simulink model "acausalFiltering_t6"  (R2012b)
settings: Solver=FixedStepDiscrete  StartTime=0.0  StopTime=10.0  FixedStep=0.001  RelTol=1e-3
undefined symbols (not defined in the file): dfilt
libraries: dspmlti4 x2, dsparch4 x2
settings Model: BufferReuse=off  Creator=gilja  LastModifiedBy=NPTL
settings SolverCC: EnableConcurrentExecution=on  ConcurrentTasks=on
settings DataIOCC: SaveOutput=off  SignalLogging=off  DSMLogging=off  SaveTime=off
settings OptimizationCC: InlineParams=on  InlineInvariantSignals=on  OptimizeBlockIOStorage=off  BufferReuse=off  ExpressionFolding=off  LocalBlockOutputs=off
settings HardwareCC: ProdIntDivRoundTo=Zero  ProdEndianess=LittleEndian  ProdHWDeviceType=Generic->32-bit x86 compatible
settings ModelReferenceCC: ModelReferenceMinAlgLoopOccurrences=on
settings RTWCC: SystemTargetFile=xpctarget.tlc  TemplateMakefile=xpc_default_tmf  Description=xPC Target  ProcessScript=xpctarget_make_rtw_hook  RTWCompilerOptimization=On
settings CodeAppCC: MaxIdLength=62
settings xpcTargetCC: TargetFcnLib=ansi_tfl_table_tmw.mat  CodeReplacementLibrary=XPC_BLAS  ParMdlRefBuildCompliant=on  ConcurrentExecutionCompliant=on  CombineSignalStateStructs=off  GRTInterface=on  xPCTaskExecutionProfile=on  xPCRL32EventNumber=5000  xPCisDownloadable=off  xPCLoadParamSetFile=off  xPCConcurrentTasks=off  xPCEnableSFAnimation=off

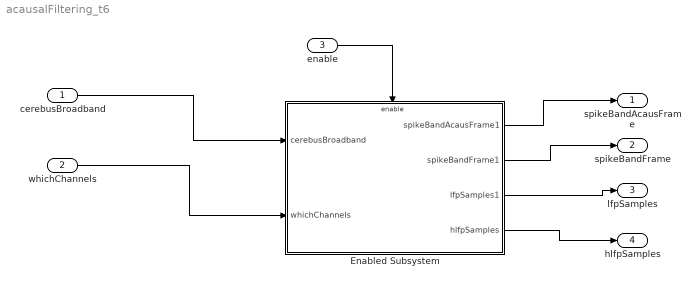
== system acausalFiltering_t6 ==
  cerebusBroadband : Inport  OutDataTypeStr=Bus: cerebusBroadband
  whichChannels : Inport  Port=2  PortDimensions=[1 32]
  enable : Inport  Port=3  OutDataTypeStr=uint8  PortDimensions=[1 1]
  Enabled Subsystem : Subsystem  TreatAsAtomicUnit=on
  spikeBandAcausFrame : Outport  BusOutputAsStruct=on
  spikeBandFrame : Outport  Port=2  BusOutputAsStruct=on
  lfpSamples : Outport  Port=3  BusOutputAsStruct=on
  hlfpSamples : Outport  Port=4  BusOutputAsStruct=on
  wires:
  cerebusBroadband/1 -> Enabled Subsystem/1(cerebusBroadband)
  whichChannels/1 -> Enabled Subsystem/2(whichChannels)
  enable/1 -> Enabled Subsystem/Enable
  Enabled Subsystem/1(spikeBandAcausFrame1) -> spikeBandAcausFrame/1
  Enabled Subsystem/2(spikeBandFrame1) -> spikeBandFrame/1
  Enabled Subsystem/3(lfpSamples1) -> lfpSamples/1
  Enabled Subsystem/4(hlfpSamples) -> hlfpSamples/1

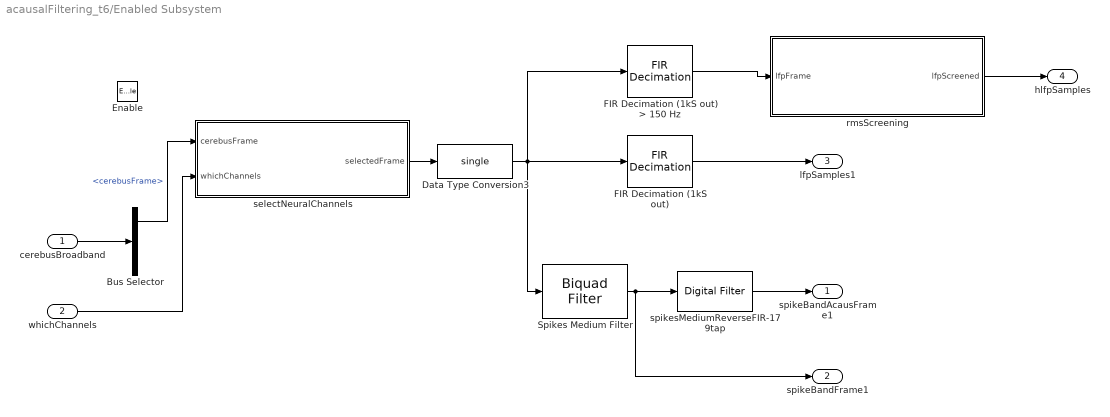
== system acausalFiltering_t6/Enabled Subsystem ==
  cerebusBroadband : Inport  OutDataTypeStr=Bus: cerebusBroadband
  whichChannels : Inport  Port=2  PortDimensions=[1 32]
  Enable : EnablePort
  Bus Selector : BusSelector  OutputSignals=cerebusFrame,outputValid,numDroppedUDPPackets
  Data Type Conversion3 : DataTypeConversion  OutDataTypeStr=single
  FIR Decimation (1kS out) : dspmlti4/FIR Decimation  h=fir1(360, 450/15000)  D=30  filtStruct=Direct form  framing=Enforce single-rate processing  inputOffset=0  outputBufInitCond=0  InputProcessing=Columns as channels (frame based)  firstCoeffDataTypeStr=Inherit: Same word length as input  firstCoeffLastDataTypeStr=Inherit: Same word length as input  firstCoeffMin=[]  firstCoeffMax=[]  outputDataTypeStr=Inherit: Same as accumulator  outputLastDataTypeStr=Inherit: Same as accumulator  outputMin=[]  outputMax=[]  roundingMode=Floor  overflowMode=off  FilterSource=Specify via dialog  FilterObject=Hm_firdecim
      settings: allowOverrides=off
  FIR Decimation (1kS out) > 150 Hz : dspmlti4/FIR Decimation  h=fir1(540, [150 450]/15000)  D=30  filtStruct=Direct form  framing=Enforce single-rate processing  inputOffset=0  outputBufInitCond=0  InputProcessing=Columns as channels (frame based)  firstCoeffDataTypeStr=Inherit: Same word length as input  firstCoeffLastDataTypeStr=Inherit: Same word length as input  firstCoeffMin=[]  firstCoeffMax=[]  outputDataTypeStr=Inherit: Same as accumulator  outputLastDataTypeStr=Inherit: Same as accumulator  outputMin=[]  outputMax=[]  roundingMode=Floor  overflowMode=off  FilterSource=Specify via dialog  FilterObject=Hm_firdecim
      settings: allowOverrides=off
  Spikes Medium Filter : dsparch4/Biquad Filter  IIRFiltStruct=Direct form II transposed  CoeffSource=Specify via dialog  BiQuadCoeffs="[0.95321773445431  -1.90644870937033 0.95323097500802 1 -1.90514144409761 0.90775595733389;  0.97970016700443  -1.95938672569874 0.97968655878878 1 -1.95804317832840 0.96073029104793]"  a0Flag=Warning  IC=0  ICnum=0  ICden=0  InputProcessing=Columns as channels (frame based)  denAccumFracLength=30  denProdOutputFracLength=30  secondMemoryFracLength=15  roundingMode=Floor  overflowMode=off  ScaleValues=1  optimizeScaleValues=on  ScaleValueMode=Specify via input port (g)  scaleValueFracLength=14  FilterSource=Specify via dialog  dfiltObjectName=dfilt.df2tsos([1 0.3 0.4],[1 0.1 0.2])
  rmsScreening : MATLAB Function  TreatAsAtomicUnit=on
  selectNeuralChannels : MATLAB Function  TreatAsAtomicUnit=on
  spikesMediumReverseFIR-179tap : dsparch4/Digital Filter  Tag=BlockMethodSubSystem  TypePopup=FIR (all zeros)  IIRFiltStruct=Direct form II transposed  AllPoleFiltStruct=Direct form  FIRFiltStruct=Direct form  CoeffSource=Specify via dialog  NumCoeffs=[0.00140028285573329 0.00145379314164095 0.00150549544372774 0.00155517517273179 0.00160261481898432 0.00164759444924944 0.00168989223087162 0.00172928498287283 0.00176554875356171 0.00179845942411888 0.00182779333752775 0.0018533279521235 0.00187484251893438 0.001892118781883 0.00190494169982069 0.00191310018925144 0.0019163878865113 0.00191460392804621 0.00190755374733714 0.00189504988690603 0.00187691282372934 0.0018529718062793 0.00182306570130567 0.00178704384836043 0.00174476691996755 0.00169610778522995 0.0016409523745676 0.00157920054317636 0.0015107669307024 0.00143558181452702 0.00135359195396933 0.00126476142262166 0.00116907242594854 0.00106652610119989 0.000957143296612834 0.000840965326803939 0.00071805470119018 0.000588495822216035 0.000452395650109955 0.000309884330846162 0.000161115783949557 6.26824674681641e-06 -0.000154455228359834 -0.000320826327031958 -0.000492591079996834 -0.000669469527359861 -0.000851155443662271 -0.00103731612710884 -0.00122759225635466 -0.0014215978181999 -0.00161892010950843 -0.00181911981658573 -0.00202173117519173 -0.0022262622142934 -0.00243219508655507 -0.00263898648845812 -0.00284606817285655 -0.00305284755660113 -0.00325870842577953 -0.00346301174092684 -0.00366509654442488 -0.0038642809721276 -0.00405986337106596 -0.00425112352489049 -0.00443732398850355 -0.0046177115331107 -0.00479151870268785 -0.00495796548265365 -0.00511626108120672 -0.00526560582364083 -0.00540519315955796 -0.00553421178272546 -0.00565184786295742 -0.00575728738913934 -0.00584971862221945 -0.00592833465663096 -0.00599233608834932 -0.00604093378741805 -0.00607335177246621 -0.00608883018440082 -0.00608662835612711 -0.00606602797479411 -0.00602633633273103 -0.00596688966289677 -0.00588705655431116 -0.00578624144260637 -0.00566388817048486 -0.00551948361255522 -0.00535256135864987 -0.00516270544943426 -0.00494955415778959 -0.00471280380912526 -0.00445221263349365 -0.00416760464208671 -0.00385887352039483 -0.00352598653007519 -0.00316898841130037 -0.00278800527713092 -0.00238324849124644 -0.00195501852016284 -0.00150370875087775 -0.00102980926475843 -0.000533910558313482 -1.6707201416282e-05 0.000520998576563121 0.00107829338229953 0.0016541492453484 0.00224742030589247 0.00285683961298849 0.0034810160428394 0.00411843134651596 0.00476743733644952 0.0054262532208052 0.00609296309471535 0.00676551359704508 0.00744171174116697 0.00811922292783734 0.0087955691479889 0.00946812738282926 0.010134128208247 0.0107906546100014 0.0114346410157853 0.0120628725495915 0.0126719845133399 0.0132584621000649 0.0138186403422851 0.0143487042986146 0.0148446894807868 0.015302482522666 0.0157178220919812 0.0160863000446657 0.0164033628209217 0.0166643130812326 0.0168643115796355 0.0169983792707087 0.0170613996457512 0.0170481212927745 0.0169531606738143 0.0167710051123323 0.0164960159823365 0.0161224320899623 0.0156443732373069 0.015055843957347 0.0143507374078498 0.0135228394112524 0.0125658326267011 0.0114733008394219 0.0102387333520141 0.00885552946126943 0.00731700300360289 0.0056163869514394 0.00374683804233694 0.00170144142218414 -0.000526784716648303 -0.00294488452160708 -0.00555995991030439 -0.00837916606463591 -0.0114097070082808 -0.0146588312871065 -0.0181338277715989 -0.0218420215999963 -0.0257907702801074 -0.0299874599670473 -0.0344395019328866 -0.0391543292432499 -0.0441393936541225 -0.0494021627406326 -0.0549501172675186 -0.0607907488087389 -0.0669315576212956 -0.0733800507753019 -0.0801437405394538 -0.0872301430174373 -0.0946467770270547 -0.102401163209666 -0.110500823353026 -0.118953279905585 -0.127766055654995 0.933868962672663]  DenCoeffs=[1 0.1]  BiQuadCoeffs=[1 0.3 0.4 1 0.1 0.2]  LatticeCoeffs=[0.2 0.4]  denIgnore=on  FiltPerSampPopup=One filter per frame  IC=0  ICnum=0  ICden=0  roundingMode=Floor  overflowMode=off  ScaleValues=1  scaleValueFracLength=14  stageInFracLength=15  stageOutFracLength=15  FilterSource=Specify via dialog  dfiltObjectName=dfilt.dffir([1 2 1])  InputProcessing=Columns as channels (frame based)
  spikeBandAcausFrame1 : Outport  BusOutputAsStruct=on
  spikeBandFrame1 : Outport  Port=2  BusOutputAsStruct=on
  lfpSamples1 : Outport  Port=3  BusOutputAsStruct=on
  hlfpSamples : Outport  Port=4  BusOutputAsStruct=on
  wires:
  spikesMediumReverseFIR-179tap/1 -> spikeBandAcausFrame1/1
  cerebusBroadband/1 -> Bus Selector/1
  Data Type Conversion3/1 -> FIR Decimation (1kS out) > 150 Hz/1, FIR Decimation (1kS out)/1, Spikes Medium Filter/1
  Spikes Medium Filter/1 -> spikesMediumReverseFIR-179tap/1, spikeBandFrame1/1
  whichChannels/1 -> selectNeuralChannels/2(whichChannels)
  Bus Selector/1 -> selectNeuralChannels/1(cerebusFrame)  "<cerebusFrame>"
  FIR Decimation (1kS out)/1 -> lfpSamples1/1
  selectNeuralChannels/1(selectedFrame) -> Data Type Conversion3/1
  FIR Decimation (1kS out) > 150 Hz/1 -> rmsScreening/1(lfpFrame)
  rmsScreening/1(lfpScreened) -> hlfpSamples/1

== matlab function acausalFiltering_t6/Enabled Subsystem/rmsScreening ==
  data: lfpFrame input; lfpScreened output; xpcConstants parameter
function lfpScreened = rmsScreening(lfpFrame, xpcConstants)
%#codegen
persistent bufferMeanSquared;
persistent bufferIdx;
persistent bufferReady;

persistent bufferCnt;

lfpScreened = lfpFrame;

if isempty(bufferIdx)
    bufferIdx = 0;
    bufferMeanSquared = single(zeros(2, size(lfpFrame, 2)));
    bufferReady=false;
    bufferCnt = 0;
end

if (bufferCnt == xpcConstants.LFPRMSperiod)
    bufferIdx = 1 - bufferIdx;
    bufferMeanSquared(2-bufferIdx, :) = 0;
    bufferReady=true;
    bufferCnt = 0;
end

bufferMeanSquared(2-bufferIdx, :) = bufferMeanSquared(2-bufferIdx, :) + lfpFrame.^2 / xpcConstants.LFPRMSperiod; 
bufferCnt = bufferCnt+1;

rmsCuttoff = 5;
if bufferReady
    for nc = 1:size(bufferMeanSquared,2)
        if abs(lfpScreened(nc)) > sqrt(bufferMeanSquared(bufferIdx+1,nc)) * rmsCuttoff;
            lfpScreened(nc) = sign(lfpScreened(nc)) * sqrt(bufferMeanSquared(bufferIdx+1,nc)) * rmsCuttoff;
        end
    end
end

== matlab function acausalFiltering_t6/Enabled Subsystem/selectNeuralChannels ==
  data: cerebusFrame input; whichChannels input double size=[1 32]; selectedFrame output
function selectedFrame = selectNeuralChannels(cerebusFrame, whichChannels)
%#codegen
persistent selectedFrameTmp
if(isempty(selectedFrameTmp))
    selectedFrameTmp = zeros(size(cerebusFrame, 1), 32);
end

selectedFrameTmp(:,1:32) = cerebusFrame(:,whichChannels);

selectedFrame = selectedFrameTmp;
